simulink model "verify_RadiationInclinedSurface_mdl"  (R2018b)
settings: Solver=FixedStepDiscrete  StartTime=280*24*3600  StopTime=281*24*3600  FixedStep=3600  RelTol=1e-3  EnableMultiTasking=on
libraries: carnot x4
settings Model: Creator=drhf  LastModifiedBy=drhf
settings DataIOCC: LimitDataPoints=on  SaveFormat=Array  SignalLoggingSaveFormat=ModelDataLogs
settings OptimizationCC: ExpressionDepthLimit=2147483647  LifeSpan=inf
settings DebuggingCC: UnderspecifiedInitializationDetection=Classic  MergeDetectMultiDrivingBlocksExec=none  SolverPrmCheckMsg=warning  FcnCallInpInsideContextMsg=warning  StateNameClashWarn=warning  SFUnexpectedBacktrackingDiag=warning  SFNoUnconditionalDefaultTransitionDiag=warning  SFExecutionAtInitializationDiag=none
settings HardwareCC: ProdBitPerPointer=32  ProdBitPerSizeT=32  ProdBitPerPtrDiffT=32  ProdLargestAtomicFloat=None  ProdIntDivRoundTo=Undefined  ProdEndianess=Unspecified  ProdWordSize=32  ProdHWDeviceType=32-bit Generic
settings ModelReferenceCC: PropagateSignalLabelsOutOfModel=off
settings SFSimCC: SimUseLocalCustomCode=off
settings RTWCC: RTWUseLocalCustomCode=off
settings CodeAppCC: StateflowObjectComments=on
settings GRTTargetCC: TargetLangStandard=C89/C90 (ANSI)  GeneratePreprocessorConditionals=Disable all  CombineOutputUpdateFcns=off  GRTInterface=on
settings ConfigComp: CovMetricSettings=dw  CovHtmlReporting=on  CovSaveCumulativeToWorkspaceVar=on  CovSaveSingleToWorkspaceVar=on  CovExternalEMLEnable=off

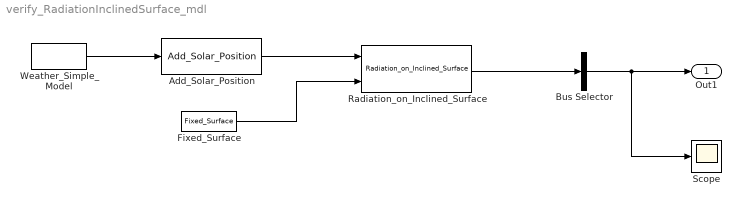
== system verify_RadiationInclinedSurface_mdl ==
  Add_Solar_Position : carnot/Weather/Add_Solar_Position  longi=0  lati=45  timezone=0
      settings: SourceProductName=Carnot
  Bus Selector : BusSelector  OutputSignals=Incidence_Angle_sun,Incidence_Angle_longitudinal,Incidence_Angle_transversal  OutputAsBus=on
  Fixed_Surface : carnot/Weather/Fixed_Surface  colangle=90  colazi=90  colrot=0
      settings: SourceProductName=Carnot
  Radiation_on_Inclined_Surface : carnot/Weather/Radiation_on_Inclined_Surface  sky=Perez 1990  reflect=0.2
      settings: SourceProductName=Carnot
  Scope : Scope
  Weather_Simple_Model : carnot/Weather/Weather_Simple_Model  lat=45  Ibn=900  Idg=100  tamb=5  deltaTsky=-6  rh=50  precip="10e-3/24/3600           % 10 mm in 24 h"  cloud=0.125  p=1013e2  vw=1  wdir=270
      settings: SourceProductName=Carnot
  Out1 : Outport
  wires:
  Weather_Simple_Model/1 -> Add_Solar_Position/1
  Bus Selector/1 -> Out1/1, Scope/1
  Fixed_Surface/1 -> Radiation_on_Inclined_Surface/2
  Add_Solar_Position/1 -> Radiation_on_Inclined_Surface/1
  Radiation_on_Inclined_Surface/1 -> Bus Selector/1
